simulink model "my_turn_pp"  (R2020a)
settings: Solver=FixedStepAuto  StartTime=0.0  StopTime=7  FixedStep=.05  RelTol=1e-3
undefined symbols (not defined in the file or in its folder): angdiff
settings Model: Creator=Jamie  LastModifiedBy=Jamie

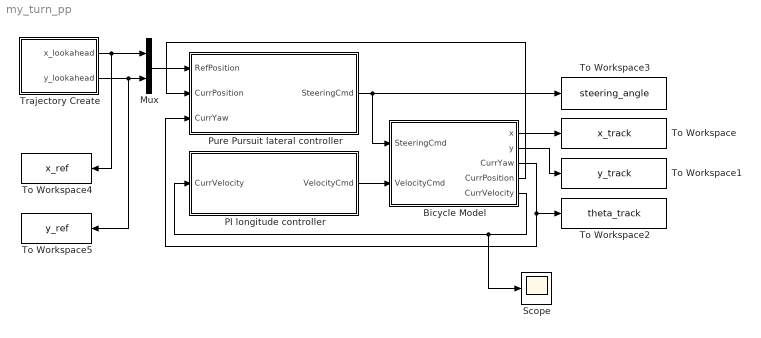
== system my_turn_pp ==
  Bicycle Model : Subsystem
  Mux : Mux  Inputs=2
  PI longitude controller : Subsystem
  "Pure Pursuit lateral controller　" : Subsystem
  Scope : Scope
  To Workspace : ToWorkspace  VariableName=x_track  SampleTime=-1
      settings: Save2DSignal=2-D array (concatenate along first dimension)
  To Workspace1 : ToWorkspace  VariableName=y_track  SampleTime=-1
      settings: Save2DSignal=2-D array (concatenate along first dimension)
  To Workspace2 : ToWorkspace  VariableName=theta_track  SampleTime=-1
      settings: Save2DSignal=2-D array (concatenate along first dimension)
  To Workspace3 : ToWorkspace  VariableName=steering_angle  SampleTime=-1
      settings: Save2DSignal=2-D array (concatenate along first dimension)
  To Workspace4 : ToWorkspace  VariableName=x_ref  SampleTime=-1
      settings: Save2DSignal=2-D array (concatenate along first dimension)
  To Workspace5 : ToWorkspace  VariableName=y_ref  SampleTime=-1
      settings: Save2DSignal=2-D array (concatenate along first dimension)
  Trajectory Create : Subsystem
  wires:
  Mux/1 -> "Pure Pursuit lateral controller　"/1(RefPosition)
  Bicycle Model/4(CurrPosition) -> "Pure Pursuit lateral controller　"/2(CurrPosition)
  "Pure Pursuit lateral controller　"/1(SteeringCmd) -> To Workspace3/1, Bicycle Model/1(SteeringCmd)
  Bicycle Model/3(CurrYaw) -> To Workspace2/1, "Pure Pursuit lateral controller　"/3(CurrYaw)
  Bicycle Model/1(x) -> To Workspace/1
  Bicycle Model/2(y) -> To Workspace1/1
  Bicycle Model/5(CurrVelocity) -> Scope/1, PI longitude controller/1(CurrVelocity)
  PI longitude controller/1(VelocityCmd) -> Bicycle Model/2(VelocityCmd)
  Trajectory Create/1(x_lookahead) -> Mux/1, To Workspace4/1
  Trajectory Create/2(y_lookahead) -> Mux/2, To Workspace5/1

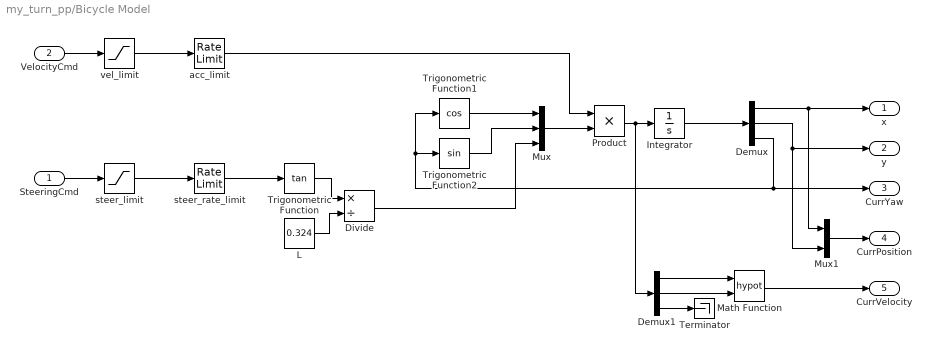
== system my_turn_pp/Bicycle Model ==
  SteeringCmd : Inport
  VelocityCmd : Inport  Port=2
  Demux : Demux  Outputs=3
  Demux1 : Demux  Outputs=3
  Divide : Product  Inputs=*/
  Integrator : Integrator  InitialCondition=[0, 0, pi/2]
  L : Constant  Value=0.324
  Math Function : Math  Operator=hypot  SaturateOnIntegerOverflow=on
  Mux : Mux  Inputs=3
  Mux1 : Mux  Inputs=2
  Product : Product
  Terminator : Terminator
  Trigonometric Function : Trigonometry  Operator=tan
  Trigonometric Function1 : Trigonometry  Operator=cos
  Trigonometric Function2 : Trigonometry
  acc_limit : RateLimiter  SampleTimeMode=inherited
  steer_limit : Saturate
  steer_rate_limit : RateLimiter  RisingSlewLimit=3  FallingSlewLimit=-3  SampleTimeMode=inherited
  vel_limit : Saturate  UpperLimit=3  LowerLimit=-3
  x : Outport
  y : Outport  Port=2
  CurrYaw : Outport  Port=3
  CurrPosition : Outport  Port=4
  CurrVelocity : Outport  Port=5
  wires:
  SteeringCmd/1 -> steer_limit/1
  VelocityCmd/1 -> vel_limit/1
  vel_limit/1 -> acc_limit/1
  steer_limit/1 -> steer_rate_limit/1
  steer_rate_limit/1 -> Trigonometric Function/1
  Trigonometric Function/1 -> Divide/1
  L/1 -> Divide/2
  acc_limit/1 -> Product/1
  Trigonometric Function1/1 -> Mux/1
  Trigonometric Function2/1 -> Mux/2
  Mux/1 -> Product/2
  Product/1 -> Demux1/1, Integrator/1
  Divide/1 -> Mux/3
  Integrator/1 -> Demux/1
  Demux/1 -> Mux1/1, x/1
  Demux/2 -> Mux1/2, y/1
  Demux/3 -> Trigonometric Function1/1, Trigonometric Function2/1, CurrYaw/1
  Mux1/1 -> CurrPosition/1
  Demux1/1 -> Math Function/1
  Demux1/2 -> Math Function/2
  Demux1/3 -> Terminator/1
  Math Function/1 -> CurrVelocity/1

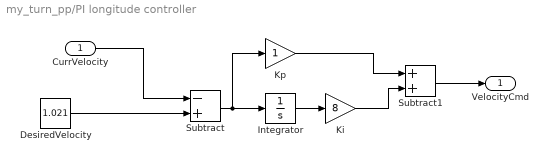
== system my_turn_pp/PI longitude controller ==
  CurrVelocity : Inport
  DesiredVelocity : Constant  Value=1.021
  Integrator : Integrator
  Ki : Gain  Gain=8
  Kp : Gain
  Subtract : Sum  Inputs=-+
  Subtract1 : Sum
  VelocityCmd : Outport
  wires:
  Subtract1/1 -> VelocityCmd/1
  DesiredVelocity/1 -> Subtract/2
  Ki/1 -> Subtract1/2
  Subtract/1 -> Integrator/1, Kp/1
  Integrator/1 -> Ki/1
  Kp/1 -> Subtract1/1
  CurrVelocity/1 -> Subtract/1

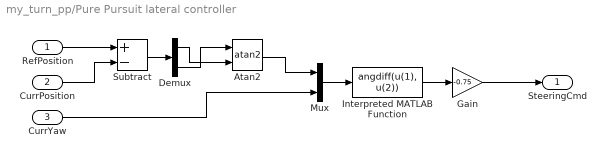
== system my_turn_pp/Pure Pursuit lateral controller　 ==
  RefPosition : Inport
  CurrPosition : Inport  Port=2
  CurrYaw : Inport  Port=3
  Atan2 : Trigonometry  Operator=atan2
  Demux : Demux  Outputs=2
  Gain : Gain  Gain=-0.75
  Interpreted MATLAB Function : MATLABFcn  MATLABFcn=angdiff(u(1), u(2))
  Mux : Mux  Inputs=2
  Subtract : Sum  Inputs=+-
  SteeringCmd : Outport
  wires:
  RefPosition/1 -> Subtract/1
  CurrPosition/1 -> Subtract/2
  Subtract/1 -> Demux/1
  Demux/2 -> Atan2/1
  Demux/1 -> Atan2/2
  Mux/1 -> Interpreted MATLAB Function/1
  Atan2/1 -> Mux/1
  CurrYaw/1 -> Mux/2
  Interpreted MATLAB Function/1 -> Gain/1
  Gain/1 -> SteeringCmd/1

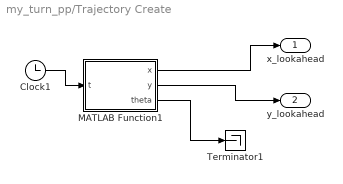
== system my_turn_pp/Trajectory Create ==
  Clock1 : Clock
  MATLAB Function1 : MATLAB Function  TreatAsAtomicUnit=on
  Terminator1 : Terminator
  x_lookahead : Outport
  y_lookahead : Outport  Port=2
  wires:
  MATLAB Function1/2(y) -> y_lookahead/1
  MATLAB Function1/1(x) -> x_lookahead/1
  Clock1/1 -> MATLAB Function1/1(t)
  MATLAB Function1/3(theta) -> Terminator1/1

== matlab function my_turn_pp/Trajectory Create/MATLAB Function1 ==
  data: x output; t input; y output; theta output
function [x, y, theta] = fcn(t)

R = 1.5;
v = 1;

if ((t >= 0)&&(t <= 1))
    x = 0;
    y = t;
    theta = 90;
elseif((t >= 1)&&(t <= 1+R*pi/v))
    x = 1.5 - 1.5*cos(v/R*(t-1));
    y = 1 + 1.5*sin(v/R*(t-1));
    theta = 90;
elseif ((t >= 1 + R*pi/v)&&(t <= 2+R*pi/v))
    x = 3;
    y = -t + 2+1.5*pi/v;
    theta = -90;
else
    x = 3;
    y = 0;
    theta = -90;
end
end
